simulink model "Fcn2"  (R2016a)
settings: Solver=VariableStepAuto  StartTime=0.0  StopTime=10.0  RelTol=1e-3
settings Model: Creator=hamza  LastModifiedBy=bourbouh

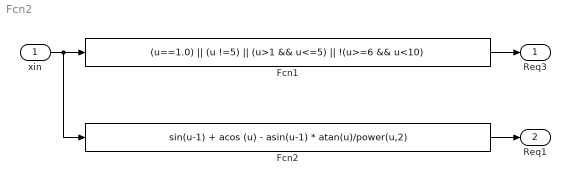
== system Fcn2 ==
  xin : Inport
  Fcn1 : Fcn  Expr=(u==1.0) || (u !=5) || (u>1 && u<=5) || !(u>=6 && u<10)
  Fcn2 : Fcn  Expr=sin(u-1) + acos (u) - asin(u-1) * atan(u)/power(u,2)
  Req3 : Outport
  Req1 : Outport  Port=2
  wires:
  Fcn1/1 -> Req3/1
  xin/1 -> Fcn2/1, Fcn1/1
  Fcn2/1 -> Req1/1
